simulink model "EPT"  (R2019b)
settings: Solver=FixedStepDiscrete  StartTime=0.0  StopTime=5  FixedStep=0.005  RelTol=1e-3  EnableMultiTasking=on
PreLoadFcn:
  | try, model_open; catch, disp('Error occurred while executing model pre-load callback: model_open.m'); disp('Please assure that the MATLAB working directory is set to the model directory before opening.'); end
InitFcn:
  | try, model_open; catch, end
undefined symbols (not defined in the file or in its folder): Bridge, GCM, H, ln, raptor_get_param_eval, raptor_get_safe_string, raptor_xcp_function
libraries: Raptor_lib x2810, simulink x374, hdlsllib x19
(part 1 of 45)
CloseFcn:
  | try, model_close; catch, end
settings Model: Raptor_Target=GCM-1793-196-1503  Raptor_Calloc=NonVolatile (EEPROM)  RaptorUIDSize=4  RaptorBuildNum=718  Raptor_ecuaddr=11  Raptor_IsLiteMode=0  Raptor_Redundant_NV=off  Raptor_Redundant_FNV=off  Creator=Ben  LastModifiedBy=user
settings SolverCC: AlgebraicLoopSolver=LineSearch
settings DataIOCC: LimitDataPoints=on  SaveFormat=Array  ReturnWorkspaceOutputs=off
settings OptimizationCC: DefaultParameterBehavior=Inlined  ExpressionDepthLimit=2147483647  InitFltsAndDblsToZero=on  LifeSpan=1  EfficientTunableParamExpr=on
settings DebuggingCC: SolverPrmCheckMsg=warning  InheritedTsInSrcMsg=none  FcnCallInpInsideContextMsg=warning  StateNameClashWarn=warning  SFUnexpectedBacktrackingDiag=warning  SFNoUnconditionalDefaultTransitionDiag=warning  SFExecutionAtInitializationDiag=none  ArithmeticOperatorsInVariantConditions=warning
settings HardwareCC: ProdBitPerPointer=32  ProdBitPerSizeT=32  ProdBitPerPtrDiffT=32  ProdLargestAtomicFloat=None  ProdWordSize=32  ProdHWDeviceType=Infineon->TriCore  TargetIntDivRoundTo=Zero  TargetEndianess=LittleEndian  ProdEqTarget=off
settings ModelReferenceCC: PropagateSignalLabelsOutOfModel=off
settings SFSimCC: SimUseLocalCustomCode=off  MATLABDynamicMemAlloc=off  CustomCodeUndefinedFunction=UseInterfaceOnly
settings RTWCC: Description=Raptor (tm)  SystemTargetFile=raptor.tlc  GenCodeOnly=on  MakeCommand=raptor_make_rtw  TemplateMakefile=raptor.tmf  RTWUseLocalCustomCode=off
settings CodeAppCC: IgnoreCustomStorageClasses=off  MaxIdLength=100  CustomSymbolStrType=$N$R$M  StateflowObjectComments=on  InternalIdentifier=Classic
settings STFCustomTargetCC: GenerateSampleERTMain=on  ModelReferenceCompliant=off  CombineOutputUpdateFcns=on  ERTCustomFileBanners=on  SupportContinuousTime=off  SupportNonInlinedSFcns=off  RemoveResetFunc=on  MATLABClassNameForMDSCustomization=Simulink.SoftwareTarget.ERTCustomization  SystemTargetFile=raptor.tlc
settings ERTTargetCC: MultiwordLength=2048  GenerateSampleERTMain=on  ModelReferenceCompliant=off  ParMdlRefBuildCompliant=off  CompOptLevelCompliant=off  ConcurrentExecutionCompliant=off  ModelStepFunctionPrototypeControlCompliant=off  CPPClassGenCompliant=off  UseToolchainInfoCompliant=off  ExtModeMexFile=noextcomm  InlinedParameterPlacement=NonHierarchical  ERTCustomFileTemplate=example_file_process.tlc  ConvertIfToSwitch=off  SuppressUnreachableDefaultCases=off
settings ConfigComp: CovMetricSettings=dw  CovHtmlReporting=on  CovSaveCumulativeToWorkspaceVar=on  CovSaveSingleToWorkspaceVar=on  CovExternalEMLEnable=off  CovSFcnEnable=off

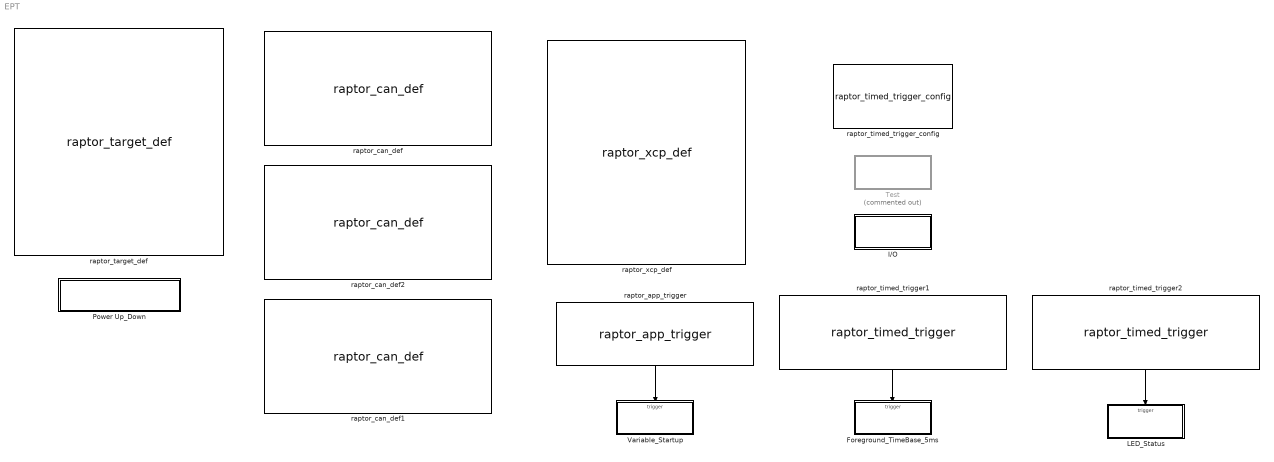
== system EPT ==
  Foreground_TimeBase_5ms : Subsystem  TreatAsAtomicUnit=on
      settings: RTWSystemCode=Nonreusable function
  I/O : Subsystem
  LED_Status : Subsystem  TreatAsAtomicUnit=on
      settings: RTWSystemCode=Nonreusable function
  Power Up_Down : Subsystem  mask{group='Diagnostics | Power Up_Down'}
  Test : Subsystem  Commented=on
  Variable_Startup : Subsystem  TreatAsAtomicUnit=on
      settings: RTWSystemCode=Nonreusable function
  raptor_app_trigger : Raptor_lib/Triggers/raptor_app_trigger  triggerValues=Startup|Shutdown|SafetyMonitor  trigger=Startup  inherited=0  alwaysEnabled=1  triggerPriority=0  triggerName=Startup_zGoy_  allowInline=0
      settings: SourceProductName=Raptor
  raptor_can_def : Raptor_lib/CAN/raptor_can_def  canBus='CAN1'  resourceValues=CAN1|CAN2|CAN3|(None)  resource=CAN1  baudRateValues=125k|250k|500k|1000k  baudRate=500k  txQueueSize=16  rxQueueSize=16
      settings: SourceProductName=Raptor
  raptor_can_def1 : Raptor_lib/CAN/raptor_can_def  canBus='CAN3'  resourceValues=CAN1|CAN2|CAN3|(None)  resource=CAN3  baudRateValues=125k|250k|500k|1000k  baudRate=500k  txQueueSize=16  rxQueueSize=16
      settings: SourceProductName=Raptor
  raptor_can_def2 : Raptor_lib/CAN/raptor_can_def  canBus='CAN2'  resourceValues=CAN1|CAN2|CAN3|(None)  resource=CAN2  baudRateValues=125k|250k|500k|1000k  baudRate=500k  txQueueSize=16  rxQueueSize=16
      settings: SourceProductName=Raptor
  raptor_target_def : Raptor_lib/Configuration/raptor_target_def  targetValues=BCM-5646-48-1404|DISP-VC128-1901|DISP-VC320L-1402|DISP-VC320-1204|DISP-VC800-1402|DISP-VC500-1904|GCM-5634M-070-1459|GCM-5634M-070-1559|GCM-5634M-070-1562|ECM-1793-196-1503|GCM-1793-196-1503|GCM-5607B-80-1901|GCM-5746R-048-1902|HCM-5534-50-1203|HCM-5534-90-1201|HCM-5534-90-1302|HCM-5534-90-1601|HCM-5534-90-1602|HCM-5604-36-1303|HCM-5604-36-1702|HCM-ARM4-070-1401|HCM-ARM4-070-1601  target=GCM-1793-196-1503  simpack=0  simulator=0  heap=4*1024  stack=2*1024  fgndStack=3*1024  bgndStack=2*1024  idleStack=1024  intStack=1536  sdStack=1024  appStack=1024  ecuaddr=11  callocValues=Constant (FLASH)|NonVolatile (EEPROM)  calloc=NonVolatile (EEPROM)  compilerValues=HighTec v3.4.5.11|HighTec v3.4.5.9  compiler=HighTec v3.4.5.11  setFileName=0  exeName=[raptor_get_safe_string(bdroot) '_']  addBuildNum=1  minVerChars=3  extraOutput=0  buildLocationValues=Raptor Default|Model Directory|User Defined  buildLocation=Raptor Default  exeLocation=''  a2lLocation=''  rpgLocation=''
      settings: SourceProductName=Raptor
  raptor_timed_trigger1 : Raptor_lib/Triggers/raptor_timed_trigger  triggerValues=Foreground|Foregroundx2|Foregroundx5|Foregroundx10|Foregroundx20|Background|Backgroundx2|Backgroundx5|Backgroundx10|Backgroundx20|Second|Minute  trigger=Foreground  inherited=0  alwaysEnabled=0  triggerPriority=0  triggerName=FGND_QFJFi
      settings: SourceProductName=Raptor
  raptor_timed_trigger2 : Raptor_lib/Triggers/raptor_timed_trigger  triggerValues=Foreground|Foregroundx2|Foregroundx5|Foregroundx10|Foregroundx20|Background|Backgroundx2|Backgroundx5|Backgroundx10|Backgroundx20|Second|Minute  trigger=Foreground  inherited=0  alwaysEnabled=0  triggerPriority=0  triggerName=FGND__22F5
      settings: SourceProductName=Raptor
  raptor_timed_trigger_config : Raptor_lib/Triggers/raptor_timed_trigger_config  triggerValues=Foreground|Background|Second|Minute  trigger=Foreground  period=5  CM2115newPeriod='RAPTOR MASK DEFAULT'
      settings: SourceProductName=Raptor
  raptor_xcp_def : Raptor_lib/Configuration/raptor_xcp_def  canBus='CAN1'  bcID=hex2dec('100')  bcID_TypeValues=Standard|Extended  bcID_Type=Standard  rxID=hex2dec('201')  rxID_TypeValues=Standard|Extended  rxID_Type=Standard  txID=hex2dec('301')  txID_TypeValues=Standard|Extended  txID_Type=Standard  daqRates=[5 10 100]  numODTs=20  genCANAPE=0  genVISION=0  securityValues=Standard|None|Custom User Defined  security=Standard  dllName=raptor_XCPSecurity.dll  accessValues=4|3|2|1  access=1
      settings: SourceProductName=Raptor
  wires:
  raptor_timed_trigger1/1 -> Foreground_TimeBase_5ms/Trigger
  raptor_app_trigger/1 -> Variable_Startup/Trigger
  raptor_timed_trigger2/1 -> LED_Status/Trigger

== system EPT/Foreground_TimeBase_5ms ==
  function : TriggerPort  TriggerType=function-call  VariantControl=Variant
  CAN : Subsystem
  CHG/DCHG_PW_Control : Subsystem
  Delay : Subsystem
  "E/W " : Subsystem
  Internal_Measurement : Subsystem
  NOT : Logic  Operator=NOT  IconShape=distinctive  AllPortsSameDT=off  OutDataTypeStr=boolean
  NOT1 : Logic  Operator=NOT  IconShape=distinctive  AllPortsSameDT=off  OutDataTypeStr=boolean
  OBP_Temp_Detection : Subsystem
  Oil/Water/Pack Cooling System : Subsystem
  System Initial : Subsystem
  System Setup : Subsystem
  SystemStart : Subsystem  TreatAsAtomicUnit=on
  raptor_adjustment8 : Raptor_lib/Data Storage/raptor_adjustment  paramName='Cal_Delay_System_Work'  nameSource=Parameter  initValue=1000  dataType=Inherit via back propagation  storage=Calibration  calDispType=Number  calEnum={'False', 'True'}  calGain=1.0  calOffset=0.0  calMax=inf  calMin=-inf  calFormat='-1'  calUnit=''  calHelp=''  calAccess=1  calFunction=raptor_xcp_function(gcb)  calDispHeaders=off  calColHeaders={'Col1' 'Col2' 'Col3'}  calRowHeaders={'Row1' 'Row2' 'Row3'}
      settings: SourceProductName=Raptor
  raptor_data_read1 : Raptor_lib/Data Storage/raptor_data_read  dataName='Flag_Ign_Off'  dataShape=Scalar  idxSource=Input  idxRow=1  idxCol=1
      settings: SourceProductName=Raptor
  raptor_data_read4 : Raptor_lib/Data Storage/raptor_data_read  dataName='Flag_Ign_Off'  dataShape=Scalar  idxSource=Input  idxRow=1  idxCol=1
      settings: SourceProductName=Raptor
  wires:
  raptor_data_read4/1 -> NOT/1
  raptor_adjustment8/1 -> Delay/2(TimeCount)
  Delay/1(Output) -> SystemStart/Trigger
  NOT/1 -> Delay/1(Condition)
  raptor_data_read1/1 -> NOT1/1, System Initial/Enable
  NOT1/1 -> CHG/DCHG_PW_Control/Enable, System Setup/Enable

== system EPT/I//O ==
  Application : Subsystem
  Input : Subsystem
  Output : Subsystem

== system EPT/LED_Status ==
  function : TriggerPort  TriggerType=function-call  VariantControl=Variant
  DualLED_Funny : Subsystem

== system EPT/Power Up_Down ==
  Background : Subsystem
  raptor_timed_trigger : Raptor_lib/Triggers/raptor_timed_trigger  triggerValues=Foreground|Foregroundx2|Foregroundx5|Foregroundx10|Foregroundx20|Background|Backgroundx2|Backgroundx5|Backgroundx10|Backgroundx20|Second|Minute  trigger=Background  inherited=0  alwaysEnabled=1  triggerPriority=50  triggerName=BGND_f_UiI
      settings: SourceProductName=Raptor
  wires:
  raptor_timed_trigger/1 -> Background/Trigger

== system EPT/Test ==
  Adjustment Variable : Subsystem  Commented=on
  Coulomb Counting Method Test : Subsystem  Commented=on
  DualLEDTest : Subsystem  Commented=on
  LED For CMU : Subsystem  Commented=on
  LifeCycleTest : Subsystem  Commented=on
  RPB1600_Read : Subsystem  Commented=on
  SINE_Wave : Subsystem  Commented=on
  Subsystem : Subsystem  Commented=on

== system EPT/Variable_Startup ==
  function : TriggerPort  TriggerType=function-call  VariantControl=Variant
  EEPROM Init : Subsystem
  Fault_init : Subsystem

== system EPT/Foreground_TimeBase_5ms/CAN ==
  CAN1_exec : Subsystem
  CAN2_exec : Subsystem
  CAN3_exec : Subsystem

== system EPT/Foreground_TimeBase_5ms/CHG//DCHG_PW_Control ==
  note: Notes:
      | IVT		:0
      | CMU	:1
  Enable : EnablePort  StatesWhenEnabling=reset
  Add : Sum
  Add1 : Sum
  Batt_Temperature Coefficient : Subsystem
  CHG/DCHG_Current_Control : Subsystem
  Coulomb Counting Algorithm : Subsystem
  Data Type Conversion{,1..3} (4 alike) : DataTypeConversion
  Demux : Demux  Outputs=2
  EOC : Subsystem
  EOD : Subsystem
  Enhanced Coulomb Counting Algorithm : Subsystem  Commented=on
  Enhanced Coulomb Counting Algorithm Backup : Subsystem  Commented=on
  Gain1 : Gain  Gain=0.5
  Gain2 : Gain  Gain=-1
  Maximum allowable Regen torque : Subsystem
  Maximum allowable torque : Subsystem
  Mux : Mux  Inputs=2
  Mux1 : Mux  Inputs=2
  PWCU PW Requirement : Subsystem
  SWU Power Divider : Subsystem
  Switch : Switch  Criteria=u2 > Threshold
  raptor_adjustment : Raptor_lib/Data Storage/raptor_adjustment  paramName='Cal_HV_DataSource'  nameSource=Parameter  initValue=0.00  dataType=double  storage=Calibration  calDispType=Number  calEnum={'False', 'True'}  calGain=1.0  calOffset=0.0  calMax=inf  calMin=-inf  calFormat='-1'  calUnit=''  calHelp=''  calAccess=1  calFunction=raptor_xcp_function(gcb)  calDispHeaders=off  calColHeaders={'Col1' 'Col2' 'Col3'}  calRowHeaders={'Row1' 'Row2' 'Row3'}
      settings: SourceProductName=Raptor
  raptor_data_def : Raptor_lib/Data Storage/raptor_data_def  dataName='EPT_BPOBU_SOC'  initValue=0  dataType=double  storage=Calibration  calVisible=on  calType=Measurement  calDispType=Number  calEnum={'False', 'True'}  calGain=1.0  calOffset=0  calMin=-inf  calMax=100  calFormat='-1'  calUnit=''  calHelp=''  calAccess=1  calFunction=raptor_xcp_function(gcb)  calDispHeaders=off  calColHeaders={'Col1' 'Col2' 'Col3'}  calRowHeaders={'Row1' 'Row2' 'Row3'}
      settings: SourceProductName=Raptor
  raptor_data_def1 : Raptor_lib/Data Storage/raptor_data_def  dataName='EPT_BPOBU_FCCAP'  initValue=0  dataType=double  storage=Volatile (RAM)  calVisible=on  calType=Measurement  calDispType=Number  calEnum={'False', 'True'}  calGain=1.0  calOffset=0  calMin=-inf  calMax=inf  calFormat='-1'  calUnit=''  calHelp=''  calAccess=1  calFunction=raptor_xcp_function(gcb)  calDispHeaders=off  calColHeaders={'Col1' 'Col2' 'Col3'}  calRowHeaders={'Row1' 'Row2' 'Row3'}
      settings: SourceProductName=Raptor
  raptor_data_def10 : Raptor_lib/Data Storage/raptor_data_def  dataName='Delta_DOD'  initValue=0  dataType=double  storage=Volatile (RAM)  calVisible=on  calType=Measurement  calDispType=Number  calEnum={'False', 'True'}  calGain=1.0  calOffset=0  calMin=-inf  calMax=inf  calFormat='-1'  calUnit=''  calHelp=''  calAccess=1  calFunction=raptor_xcp_function(gcb)  calDispHeaders=off  calColHeaders={'Col1' 'Col2' 'Col3'}  calRowHeaders={'Row1' 'Row2' 'Row3'}
      settings: SourceProductName=Raptor
  raptor_data_def11 : Raptor_lib/Data Storage/raptor_data_def  dataName='Cmax'  initValue=0  dataType=double  storage=Volatile (RAM)  calVisible=on  calType=Measurement  calDispType=Number  calEnum={'False', 'True'}  calGain=1.0  calOffset=0  calMin=-inf  calMax=inf  calFormat='-1'  calUnit=''  calHelp=''  calAccess=1  calFunction=raptor_xcp_function(gcb)  calDispHeaders=off  calColHeaders={'Col1' 'Col2' 'Col3'}  calRowHeaders={'Row1' 'Row2' 'Row3'}
      settings: SourceProductName=Raptor
  raptor_data_def12 : Raptor_lib/Data Storage/raptor_data_def  dataName='SOC'  initValue=0  dataType=double  storage=Volatile (RAM)  calVisible=on  calType=Measurement  calDispType=Number  calEnum={'False', 'True'}  calGain=1.0  calOffset=0  calMin=-inf  calMax=inf  calFormat='-1'  calUnit=''  calHelp=''  calAccess=1  calFunction=raptor_xcp_function(gcb)  calDispHeaders=off  calColHeaders={'Col1' 'Col2' 'Col3'}  calRowHeaders={'Row1' 'Row2' 'Row3'}
      settings: SourceProductName=Raptor
  raptor_data_def13 : Raptor_lib/Data Storage/raptor_data_def  dataName='SOH'  initValue=100  dataType=double  storage=Volatile (RAM)  calVisible=on  calType=Measurement  calDispType=Number  calEnum={'False', 'True'}  calGain=1.0  calOffset=0  calMin=-inf  calMax=inf  calFormat='-1'  calUnit=''  calHelp=''  calAccess=1  calFunction=raptor_xcp_function(gcb)  calDispHeaders=off  calColHeaders={'Col1' 'Col2' 'Col3'}  calRowHeaders={'Row1' 'Row2' 'Row3'}
      settings: SourceProductName=Raptor
  raptor_data_def14 : Raptor_lib/Data Storage/raptor_data_def  dataName='EPT_BPOBU_VOLT'  initValue=0  dataType=double  storage=Calibration  calVisible=on  calType=Measurement  calDispType=Number  calEnum={'False', 'True'}  calGain=1.0  calOffset=0  calMin=-inf  calMax=inf  calFormat='-1'  calUnit=''  calHelp=''  calAccess=1  calFunction=raptor_xcp_function(gcb)  calDispHeaders=off  calColHeaders={'Col1' 'Col2' 'Col3'}  calRowHeaders={'Row1' 'Row2' 'Row3'}
      settings: SourceProductName=Raptor
  raptor_data_def15 : Raptor_lib/Data Storage/raptor_data_def  dataName='DOD_t'  initValue=0  dataType=double  storage=Volatile (RAM)  calVisible=on  calType=Measurement  calDispType=Number  calEnum={'False', 'True'}  calGain=1.0  calOffset=0  calMin=-inf  calMax=inf  calFormat='-1'  calUnit=''  calHelp=''  calAccess=1  calFunction=raptor_xcp_function(gcb)  calDispHeaders=off  calColHeaders={'Col1' 'Col2' 'Col3'}  calRowHeaders={'Row1' 'Row2' 'Row3'}
      settings: SourceProductName=Raptor
  raptor_data_def2 : Raptor_lib/Data Storage/raptor_data_def  dataName='EPT_HV_BUS_VOLT'  initValue=0  dataType=double  storage=Calibration  calVisible=on  calType=Measurement  calDispType=Number  calEnum={'False', 'True'}  calGain=1.0  calOffset=0  calMin=-inf  calMax=inf  calFormat='-1'  calUnit=''  calHelp=''  calAccess=1  calFunction=raptor_xcp_function(gcb)  calDispHeaders=off  calColHeaders={'Col1' 'Col2' 'Col3'}  calRowHeaders={'Row1' 'Row2' 'Row3'}
      settings: SourceProductName=Raptor
  raptor_data_def3 : Raptor_lib/Data Storage/raptor_data_def  dataName='EPT_BPOBU_AH_DEF'  initValue=0  dataType=uint8  storage=Volatile (RAM)  calVisible=on  calType=Measurement  calDispType=Number  calEnum={'False', 'True'}  calGain=1.0  calOffset=0  calMin=-inf  calMax=inf  calFormat='-1'  calUnit=''  calHelp=''  calAccess=1  calFunction=raptor_xcp_function(gcb)  calDispHeaders=off  calColHeaders={'Col1' 'Col2' 'Col3'}  calRowHeaders={'Row1' 'Row2' 'Row3'}
      settings: SourceProductName=Raptor
  raptor_data_def4 : Raptor_lib/Data Storage/raptor_data_def  dataName='EPT_BPOBU_RCAP'  initValue=0  dataType=double  storage=Volatile (RAM)  calVisible=on  calType=Measurement  calDispType=Number  calEnum={'False', 'True'}  calGain=1.0  calOffset=0  calMin=-inf  calMax=150  calFormat='-1'  calUnit=''  calHelp=''  calAccess=1  calFunction=raptor_xcp_function(gcb)  calDispHeaders=off  calColHeaders={'Col1' 'Col2' 'Col3'}  calRowHeaders={'Row1' 'Row2' 'Row3'}
      settings: SourceProductName=Raptor
  raptor_data_def5 : Raptor_lib/Data Storage/raptor_data_def  dataName='EPT_BPOBU_SOA'  initValue=1  dataType=double  storage=Volatile (RAM)  calVisible=on  calType=Measurement  calDispType=Number  calEnum={'False', 'True'}  calGain=1.0  calOffset=0  calMin=-inf  calMax=inf  calFormat='-1'  calUnit=''  calHelp=''  calAccess=1  calFunction=raptor_xcp_function(gcb)  calDispHeaders=off  calColHeaders={'Col1' 'Col2' 'Col3'}  calRowHeaders={'Row1' 'Row2' 'Row3'}
      settings: SourceProductName=Raptor
  raptor_data_def6 : Raptor_lib/Data Storage/raptor_data_def  dataName='EPT_HV_LEAK_VOLT'  initValue=0  dataType=double  storage=Calibration  calVisible=on  calType=Measurement  calDispType=Number  calEnum={'False', 'True'}  calGain=1.0  calOffset=0  calMin=-inf  calMax=inf  calFormat='-1'  calUnit=''  calHelp=''  calAccess=1  calFunction=raptor_xcp_function(gcb)  calDispHeaders=off  calColHeaders={'Col1' 'Col2' 'Col3'}  calRowHeaders={'Row1' 'Row2' 'Row3'}
      settings: SourceProductName=Raptor
  raptor_data_def7 : Raptor_lib/Data Storage/raptor_data_def  dataName='EPT_BPOBU_CURR'  initValue=0  dataType=double  storage=Calibration  calVisible=on  calType=Measurement  calDispType=Number  calEnum={'False', 'True'}  calGain=1.0  calOffset=0  calMin=-inf  calMax=inf  calFormat='-1'  calUnit=''  calHelp=''  calAccess=1  calFunction=raptor_xcp_function(gcb)  calDispHeaders=off  calColHeaders={'Col1' 'Col2' 'Col3'}  calRowHeaders={'Row1' 'Row2' 'Row3'}
      settings: SourceProductName=Raptor
  raptor_data_def8 : Raptor_lib/Data Storage/raptor_data_def  dataName='New_SOH'  initValue=100  dataType=double  storage=Volatile (RAM)  calVisible=on  calType=Measurement  calDispType=Number  calEnum={'False', 'True'}  calGain=1.0  calOffset=0  calMin=-inf  calMax=inf  calFormat='-1'  calUnit=''  calHelp=''  calAccess=1  calFunction=raptor_xcp_function(gcb)  calDispHeaders=off  calColHeaders={'Col1' 'Col2' 'Col3'}  calRowHeaders={'Row1' 'Row2' 'Row3'}
      settings: SourceProductName=Raptor
  raptor_data_def9 : Raptor_lib/Data Storage/raptor_data_def  dataName='DOD_t0'  initValue=0  dataType=double  storage=Volatile (RAM)  calVisible=on  calType=Measurement  calDispType=Number  calEnum={'False', 'True'}  calGain=1.0  calOffset=0  calMin=-inf  calMax=inf  calFormat='-1'  calUnit=''  calHelp=''  calAccess=1  calFunction=raptor_xcp_function(gcb)  calDispHeaders=off  calColHeaders={'Col1' 'Col2' 'Col3'}  calRowHeaders={'Row1' 'Row2' 'Row3'}
      settings: SourceProductName=Raptor
  raptor_data_read1 : Raptor_lib/Data Storage/raptor_data_read  dataName='CMU2_BATT_CURR'  dataShape=Scalar  idxSource=Input  idxRow=1  idxCol=1
      settings: SourceProductName=Raptor
  raptor_data_read10 : Raptor_lib/Data Storage/raptor_data_read  dataName='I_Current'  dataShape=Scalar  idxSource=Input  idxRow=1  idxCol=1
      settings: SourceProductName=Raptor
  raptor_data_read11 : Raptor_lib/Data Storage/raptor_data_read  dataName='U1_Voltage'  dataShape=Scalar  idxSource=Input  idxRow=1  idxCol=1
      settings: SourceProductName=Raptor
  raptor_data_read12 : Raptor_lib/Data Storage/raptor_data_read  dataName='U2_Voltage'  dataShape=Scalar  idxSource=Input  idxRow=1  idxCol=1
      settings: SourceProductName=Raptor
  raptor_data_read13 : Raptor_lib/Data Storage/raptor_data_read  dataName='U3_Voltage'  dataShape=Scalar  idxSource=Input  idxRow=1  idxCol=1
      settings: SourceProductName=Raptor
  raptor_data_read2 : Raptor_lib/Data Storage/raptor_data_read  dataName='CMU1_BATT_CURR'  dataShape=Scalar  idxSource=Input  idxRow=1  idxCol=1
      settings: SourceProductName=Raptor
  raptor_data_read4 : Raptor_lib/Data Storage/raptor_data_read  dataName='CMU2_BATT_VOLT'  dataShape=Scalar  idxSource=Input  idxRow=1  idxCol=1
      settings: SourceProductName=Raptor
  raptor_data_read7 : Raptor_lib/Data Storage/raptor_data_read  dataName='CMU1_BATT_VOLT'  dataShape=Scalar  idxSource=Input  idxRow=1  idxCol=1
      settings: SourceProductName=Raptor
  raptor_data_write1 : Raptor_lib/Data Storage/raptor_data_write  dataName='EPT_BPOBU_CURR'  dataShape=Scalar  idxSource=Input Port  idxRow=1  idxCol=1
      settings: SourceProductName=Raptor
  raptor_data_write2 : Raptor_lib/Data Storage/raptor_data_write  dataName='EPT_BPOBU_VOLT'  dataShape=Scalar  idxSource=Input Port  idxRow=1  idxCol=1
      settings: SourceProductName=Raptor
  raptor_data_write4 : Raptor_lib/Data Storage/raptor_data_write  dataName='EPT_HV_BUS_VOLT'  dataShape=Scalar  idxSource=Input Port  idxRow=1  idxCol=1
      settings: SourceProductName=Raptor
  raptor_data_write5 : Raptor_lib/Data Storage/raptor_data_write  dataName='EPT_HV_LEAK_VOLT'  dataShape=Scalar  idxSource=Input Port  idxRow=1  idxCol=1
      settings: SourceProductName=Raptor
  wires:
  Batt_Temperature Coefficient/1(Ft) -> CHG/DCHG_Current_Control/1(Ft)
  raptor_data_read4/1 -> Add/2
  raptor_data_read7/1 -> Add/1
  CHG/DCHG_Current_Control/1(Idchg_exp) -> Maximum allowable torque/1(Idchg_con)
  Add1/1 -> Gain1/1
  raptor_data_read2/1 -> Add1/1
  raptor_data_read1/1 -> Add1/2
  CHG/DCHG_Current_Control/2(Iregen_con) -> Maximum allowable Regen torque/1(Iregen_con)
  Mux/1 -> Switch/3
  raptor_data_read10/1 -> Data Type Conversion/1
  raptor_data_read11/1 -> Data Type Conversion1/1
  Switch/1 -> Demux/1
  Gain1/1 -> Mux1/1
  Add/1 -> Mux1/2
  Mux1/1 -> Switch/1
  Demux/1 -> raptor_data_write1/1
  Demux/2 -> raptor_data_write2/1
  Data Type Conversion/1 -> Gain2/1
  Data Type Conversion1/1 -> Mux/2
  raptor_adjustment/1 -> Switch/2
  raptor_data_read12/1 -> Data Type Conversion2/1
  raptor_data_read13/1 -> Data Type Conversion3/1
  Data Type Conversion2/1 -> raptor_data_write4/1
  Data Type Conversion3/1 -> raptor_data_write5/1
  Gain2/1 -> Mux/1

== system EPT/Foreground_TimeBase_5ms/Delay ==
  Condition : Inport
  TimeCount : Inport  Port=2
  Constant10 : Constant
  Constant11 : Constant  Value=0
  Constant8 : Constant  Value=0
  CycleTrigger : Subsystem
  Switch2 : Switch  Threshold=1
  Switch3 : Switch  Threshold=1
  Unit Delay1 : UnitDelay  SampleTime=-1  HasFrameUpgradeWarning=on
  Unit Delay3 : UnitDelay  SampleTime=-1  HasFrameUpgradeWarning=on
  Output : Outport  VectorParamsAs1DForOutWhenUnconnected=off
  wires:
  TimeCount/1 -> CycleTrigger/2(In2)
  Condition/1 -> Switch3/2
  Constant8/1 -> Switch2/1
  CycleTrigger/1(Trigger) -> Switch2/2, Unit Delay3/1
  Constant10/1 -> Switch2/3
  Switch3/1 -> CycleTrigger/1(In1)
  Switch2/1 -> Unit Delay1/1
  Constant11/1 -> Switch3/3
  Unit Delay1/1 -> Switch3/1
  Unit Delay3/1 -> Output/1

== system EPT/Foreground_TimeBase_5ms/E//W  ==
  BP-OBU_E/W : Subsystem
  CAN_E/W : Subsystem
  E/W_Process : Subsystem

== system EPT/Foreground_TimeBase_5ms/Internal_Measurement ==
  raptor_data_def1 : Raptor_lib/Data Storage/raptor_data_def  dataName='Sensor_5V_Volt'  initValue=0  dataType=double  storage=Volatile (RAM)  calVisible=on  calType=Measurement  calDispType=Number  calEnum={'False', 'True'}  calGain=1.0  calOffset=0  calMin=-inf  calMax=inf  calFormat='-1'  calUnit=''  calHelp=''  calAccess=1  calFunction=raptor_xcp_function(gcb)  calDispHeaders=off  calColHeaders={'Col1' 'Col2' 'Col3'}  calRowHeaders={'Row1' 'Row2' 'Row3'}
      settings: SourceProductName=Raptor
  raptor_data_def4 : Raptor_lib/Data Storage/raptor_data_def  dataName='I2V_Battery_Volt'  initValue=0  dataType=double  storage=Volatile (RAM)  calVisible=on  calType=Measurement  calDispType=Number  calEnum={'False', 'True'}  calGain=1.0  calOffset=0  calMin=-inf  calMax=inf  calFormat='-1'  calUnit=''  calHelp=''  calAccess=1  calFunction=raptor_xcp_function(gcb)  calDispHeaders=off  calColHeaders={'Col1' 'Col2' 'Col3'}  calRowHeaders={'Row1' 'Row2' 'Row3'}
      settings: SourceProductName=Raptor
  raptor_data_write1 : Raptor_lib/Data Storage/raptor_data_write  dataName='Sensor_5V_Volt'  dataShape=Scalar  idxSource=Input Port  idxRow=1  idxCol=1
      settings: SourceProductName=Raptor
  raptor_data_write2 : Raptor_lib/Data Storage/raptor_data_write  dataName='I2V_Battery_Volt'  dataShape=Scalar  idxSource=Input Port  idxRow=1  idxCol=1
      settings: SourceProductName=Raptor
  raptor_internal_measurement : Raptor_lib/Input & Output/raptor_internal_measurement  resourceValues=BATTERY_VOLTAGE|VSENS_SUPPLY|LAST_RESET|RESET_CNT|(None)  resource=BATTERY_VOLTAGE  out_eng=1  soft_filter=1  out_bool=0
      settings: SourceProductName=Raptor
  raptor_internal_measurement1 : Raptor_lib/Input & Output/raptor_internal_measurement  resourceValues=BATTERY_VOLTAGE|VSENS_SUPPLY|LAST_RESET|RESET_CNT|(None)  resource=VSENS_SUPPLY  out_eng=1  soft_filter=1  out_bool=0
      settings: SourceProductName=Raptor
  raptor_internal_measurement2 : Raptor_lib/Input & Output/raptor_internal_measurement  resourceValues=BATTERY_VOLTAGE|VSENS_SUPPLY|LAST_RESET|RESET_CNT|(None)  resource=LAST_RESET  out_eng=1  soft_filter=1  out_bool=0
      settings: SourceProductName=Raptor
  raptor_internal_measurement3 : Raptor_lib/Input & Output/raptor_internal_measurement  resourceValues=BATTERY_VOLTAGE|VSENS_SUPPLY|LAST_RESET|RESET_CNT|(None)  resource=RESET_CNT  out_eng=1  soft_filter=1  out_bool=0
      settings: SourceProductName=Raptor
  raptor_measurement2 : Raptor_lib/Data Storage/raptor_measurement  paramName='Last_Reset'  nameSource=Parameter  calDispType=Number  calEnum={'False', 'True'}  calGain=1.0  calOffset=0.0  calMax=inf  calMin=-inf  calFormat='-1'  calUnit=''  calHelp=''  calAccess=1  calFunction=raptor_xcp_function(gcb)  calVisible=on
      settings: SourceProductName=Raptor
  raptor_measurement3 : Raptor_lib/Data Storage/raptor_measurement  paramName='Reset_CNT'  nameSource=Parameter  calDispType=Number  calEnum={'False', 'True'}  calGain=1.0  calOffset=0.0  calMax=inf  calMin=-inf  calFormat='-1'  calUnit=''  calHelp=''  calAccess=1  calFunction=raptor_xcp_function(gcb)  calVisible=on
      settings: SourceProductName=Raptor
  wires:
  raptor_internal_measurement/1 -> raptor_data_write2/1
  raptor_internal_measurement3/1 -> raptor_measurement3/1
  raptor_internal_measurement2/1 -> raptor_measurement2/1
  raptor_internal_measurement1/1 -> raptor_data_write1/1

== system EPT/Foreground_TimeBase_5ms/OBP_Temp_Detection ==
  ADC2Degree : Subsystem
  Constant2 : Constant  Value=20
  CountTrigger : Subsystem
  wires:
  CountTrigger/1(Tirgger) -> ADC2Degree/Trigger
  Constant2/1 -> CountTrigger/1(Counter)

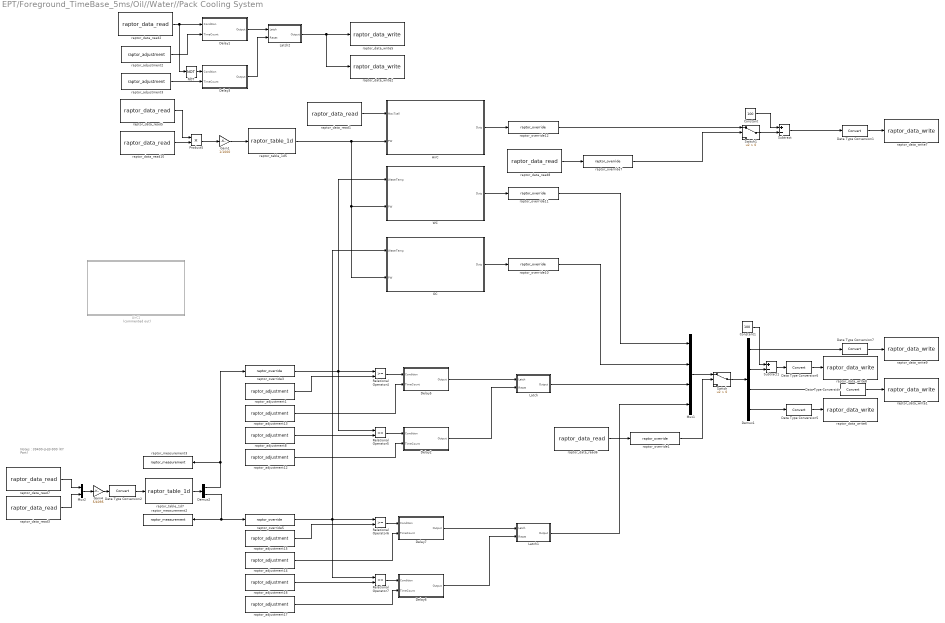
== system EPT/Foreground_TimeBase_5ms/Oil//Water//Pack Cooling System ==
  note: Notes :
      | 39400-LHJ3-900
      | (KY Part)
  AirC : Subsystem
  AirC1 : Subsystem  Commented=on
  Constant : Constant  Value=100
  Constant1 : Constant  Value=100
  Data Type Conversion{,1..2,5..7} (6 alike) : DataTypeConversion
  Delay1 : Subsystem
  Delay2 : Subsystem
  Delay3 : Subsystem
  Delay5 : Subsystem
  Delay6 : Subsystem
  Delay7 : Subsystem
  Demux1 : Demux
  Demux2 : Demux  Outputs=2
  Gain1 : Gain  Gain=1/1000
  Gain4 : Gain  Gain=5/4095
  Latch : Subsystem
  Latch1 : Subsystem
  Latch2 : Subsystem
  Mux1 : Mux
  Mux2 : Mux  Inputs=2
  NOT : Logic  Operator=NOT  IconShape=distinctive  AllPortsSameDT=off  OutDataTypeStr=boolean
  OC : Subsystem
  Product5 : Product
  Relational Operator4 : RelationalOperator  OutDataTypeStr=boolean  RndMeth=Simplest
  Relational Operator5 : RelationalOperator  Operator=<=  OutDataTypeStr=boolean  RndMeth=Simplest
  Relational Operator6 : RelationalOperator  OutDataTypeStr=boolean  RndMeth=Simplest
  Relational Operator7 : RelationalOperator  Operator=<=  OutDataTypeStr=boolean  RndMeth=Simplest
  Subtract : Sum  Inputs=+-
  Subtract1 : Sum  Inputs=+-
  Switch : Switch  Criteria=u2 > Threshold
  Switch1 : Switch  Criteria=u2 > Threshold
  WC : Subsystem
  raptor_adjustment1 : Raptor_lib/Data Storage/raptor_adjustment  paramName='Cal_Cooling_Water_Temp_LimitHigh'  nameSource=Parameter  initValue=55  dataType=double  storage=Calibration  calDispType=Number  calEnum={'False', 'True'}  calGain=1.0  calOffset=0.0  calMax=inf  calMin=-inf  calFormat='-1'  calUnit=''  calHelp=''  calAccess=1  calFunction=raptor_xcp_function(gcb)  calDispHeaders=off  calColHeaders={'Col1' 'Col2' 'Col3'}  calRowHeaders={'Row1' 'Row2' 'Row3'}
      settings: SourceProductName=Raptor
  raptor_adjustment12 : Raptor_lib/Data Storage/raptor_adjustment  paramName='Cal_Water_Cooling_Fan_Off_DelayTime'  nameSource=Parameter  initValue=1000  dataType=double  storage=Calibration  calDispType=Number  calEnum={'False', 'True'}  calGain=1.0  calOffset=0.0  calMax=inf  calMin=-inf  calFormat='-1'  calUnit=''  calHelp=''  calAccess=1  calFunction=raptor_xcp_function(gcb)  calDispHeaders=off  calColHeaders={'Col1' 'Col2' 'Col3'}  calRowHeaders={'Row1' 'Row2' 'Row3'}
      settings: SourceProductName=Raptor
  raptor_adjustment13 : Raptor_lib/Data Storage/raptor_adjustment  paramName='Cal_Water_Cooling_Fan_On_DelayTime'  nameSource=Parameter  initValue=0.00  dataType=double  storage=Calibration  calDispType=Number  calEnum={'False', 'True'}  calGain=1.0  calOffset=0.0  calMax=inf  calMin=-inf  calFormat='-1'  calUnit=''  calHelp=''  calAccess=1  calFunction=raptor_xcp_function(gcb)  calDispHeaders=off  calColHeaders={'Col1' 'Col2' 'Col3'}  calRowHeaders={'Row1' 'Row2' 'Row3'}
      settings: SourceProductName=Raptor
  raptor_adjustment14 : Raptor_lib/Data Storage/raptor_adjustment  paramName='Cal_Oil_Cooling_Fan_On_DelayTime'  nameSource=Parameter  initValue=0.00  dataType=double  storage=Calibration  calDispType=Number  calEnum={'False', 'True'}  calGain=1.0  calOffset=0.0  calMax=inf  calMin=-inf  calFormat='-1'  calUnit=''  calHelp=''  calAccess=1  calFunction=raptor_xcp_function(gcb)  calDispHeaders=off  calColHeaders={'Col1' 'Col2' 'Col3'}  calRowHeaders={'Row1' 'Row2' 'Row3'}
      settings: SourceProductName=Raptor
  raptor_adjustment15 : Raptor_lib/Data Storage/raptor_adjustment  paramName='Cal_Cooling_Oil_Temp_LimitHigh'  nameSource=Parameter  initValue=70  dataType=double  storage=Calibration  calDispType=Number  calEnum={'False', 'True'}  calGain=1.0  calOffset=0.0  calMax=inf  calMin=-inf  calFormat='-1'  calUnit=''  calHelp=''  calAccess=1  calFunction=raptor_xcp_function(gcb)  calDispHeaders=off  calColHeaders={'Col1' 'Col2' 'Col3'}  calRowHeaders={'Row1' 'Row2' 'Row3'}
      settings: SourceProductName=Raptor
  raptor_adjustment16 : Raptor_lib/Data Storage/raptor_adjustment  paramName='Cal_Cooling_Oil_Temp_LimitLow'  nameSource=Parameter  initValue=60  dataType=double  storage=Calibration  calDispType=Number  calEnum={'False', 'True'}  calGain=1.0  calOffset=0.0  calMax=inf  calMin=-inf  calFormat='-1'  calUnit=''  calHelp=''  calAccess=1  calFunction=raptor_xcp_function(gcb)  calDispHeaders=off  calColHeaders={'Col1' 'Col2' 'Col3'}  calRowHeaders={'Row1' 'Row2' 'Row3'}
      settings: SourceProductName=Raptor
  raptor_adjustment17 : Raptor_lib/Data Storage/raptor_adjustment  paramName='Cal_Oil_Cooling_Fan_Off_DelayTime'  nameSource=Parameter  initValue=3000  dataType=double  storage=Calibration  calDispType=Number  calEnum={'False', 'True'}  calGain=1.0  calOffset=0.0  calMax=inf  calMin=-inf  calFormat='-1'  calUnit=''  calHelp=''  calAccess=1  calFunction=raptor_xcp_function(gcb)  calDispHeaders=off  calColHeaders={'Col1' 'Col2' 'Col3'}  calRowHeaders={'Row1' 'Row2' 'Row3'}
      settings: SourceProductName=Raptor
  raptor_adjustment2 : Raptor_lib/Data Storage/raptor_adjustment  paramName='Cal_EAU_On_DelayTime'  nameSource=Parameter  initValue=0.00  dataType=double  storage=Calibration  calDispType=Number  calEnum={'False', 'True'}  calGain=1.0  calOffset=0.0  calMax=inf  calMin=-inf  calFormat='-1'  calUnit=''  calHelp=''  calAccess=1  calFunction=raptor_xcp_function(gcb)  calDispHeaders=off  calColHeaders={'Col1' 'Col2' 'Col3'}  calRowHeaders={'Row1' 'Row2' 'Row3'}
      settings: SourceProductName=Raptor
  raptor_adjustment3 : Raptor_lib/Data Storage/raptor_adjustment  paramName='Cal_EAU_Off_DelayTime'  nameSource=Parameter  initValue=100  dataType=double  storage=Calibration  calDispType=Number  calEnum={'False', 'True'}  calGain=1.0  calOffset=0.0  calMax=inf  calMin=-inf  calFormat='-1'  calUnit=''  calHelp=''  calAccess=1  calFunction=raptor_xcp_function(gcb)  calDispHeaders=off  calColHeaders={'Col1' 'Col2' 'Col3'}  calRowHeaders={'Row1' 'Row2' 'Row3'}
      settings: SourceProductName=Raptor
  raptor_adjustment8 : Raptor_lib/Data Storage/raptor_adjustment  paramName='Cal_Cooling_Water_Temp_LimitLow'  nameSource=Parameter  initValue=50  dataType=double  storage=Calibration  calDispType=Number  calEnum={'False', 'True'}  calGain=1.0  calOffset=0.0  calMax=inf  calMin=-inf  calFormat='-1'  calUnit=''  calHelp=''  calAccess=1  calFunction=raptor_xcp_function(gcb)  calDispHeaders=off  calColHeaders={'Col1' 'Col2' 'Col3'}  calRowHeaders={'Row1' 'Row2' 'Row3'}
      settings: SourceProductName=Raptor
  raptor_data_read1 : Raptor_lib/Data Storage/raptor_data_read  dataName='Max_CellT'  dataShape=Scalar  idxSource=Input  idxRow=1  idxCol=1
      settings: SourceProductName=Raptor
  raptor_data_read10 : Raptor_lib/Data Storage/raptor_data_read  dataName='EPT_BPOBU_VOLT'  dataShape=Scalar  idxSource=Input  idxRow=1  idxCol=1
      settings: SourceProductName=Raptor
  raptor_data_read2 : Raptor_lib/Data Storage/raptor_data_read  dataName='Relay_DCDC_12V'  dataShape=Scalar  idxSource=Input  idxRow=1  idxCol=1
      settings: SourceProductName=Raptor
  raptor_data_read3 : Raptor_lib/Data Storage/raptor_data_read  dataName='A105_Cooling_Oil_Temp_in'  dataShape=Scalar  idxSource=Input  idxRow=1  idxCol=1
      settings: SourceProductName=Raptor
  raptor_data_read5 : Raptor_lib/Data Storage/raptor_data_read  dataName='EPT_BPOBU_CURR'  dataShape=Scalar  idxSource=Input  idxRow=1  idxCol=1
      settings: SourceProductName=Raptor
  raptor_data_read6 : Raptor_lib/Data Storage/raptor_data_read  dataName='K37_LSD_Relay_EAU1'  dataShape=Scalar  idxSource=Input  idxRow=1  idxCol=1
      settings: SourceProductName=Raptor
  raptor_data_read7 : Raptor_lib/Data Storage/raptor_data_read  dataName='A17_Cooling_Water_Temp_in'  dataShape=Scalar  idxSource=Input  idxRow=1  idxCol=1
      settings: SourceProductName=Raptor
  raptor_data_read8 : Raptor_lib/Data Storage/raptor_data_read  dataName='K19_LSD_Relay_EAU2'  dataShape=Scalar  idxSource=Input  idxRow=1  idxCol=1
      settings: SourceProductName=Raptor
  raptor_data_write1 : Raptor_lib/Data Storage/raptor_data_write  dataName='K55_LSD_Relay_WC'  dataShape=Scalar  idxSource=Input Port  idxRow=1  idxCol=1
      settings: SourceProductName=Raptor
  raptor_data_write2 : Raptor_lib/Data Storage/raptor_data_write  dataName='K19_LSD_Relay_EAU2'  dataShape=Scalar  idxSource=Input Port  idxRow=1  idxCol=1
      settings: SourceProductName=Raptor
  raptor_data_write5 : Raptor_lib/Data Storage/raptor_data_write  dataName='K37_LSD_Relay_EAU1'  dataShape=Scalar  idxSource=Input Port  idxRow=1  idxCol=1
      settings: SourceProductName=Raptor
  raptor_data_write6 : Raptor_lib/Data Storage/raptor_data_write  dataName='A46_LSD_Relay_OC'  dataShape=Scalar  idxSource=Input Port  idxRow=1  idxCol=1
      settings: SourceProductName=Raptor
  raptor_data_write7 : Raptor_lib/Data Storage/raptor_data_write  dataName='K88_LSD_PWM_Duty'  dataShape=Scalar  idxSource=Input Port  idxRow=1  idxCol=1
      settings: SourceProductName=Raptor
  raptor_data_write8 : Raptor_lib/Data Storage/raptor_data_write  dataName='A23_LSD_PWM_Duty'  dataShape=Scalar  idxSource=Input Port  idxRow=1  idxCol=1
      settings: SourceProductName=Raptor
  raptor_data_write9 : Raptor_lib/Data Storage/raptor_data_write  dataName='A93_LSD_PWM_Duty'  dataShape=Scalar  idxSource=Input Port  idxRow=1  idxCol=1
      settings: SourceProductName=Raptor
  raptor_measurement2 : Raptor_lib/Data Storage/raptor_measurement  paramName='Oil_Temp'  nameSource=Parameter  calDispType=Number  calEnum={'False', 'True'}  calGain=1.0  calOffset=0.0  calMax=inf  calMin=-inf  calFormat='-1'  calUnit=''  calHelp=''  calAccess=1  calFunction=raptor_xcp_function(gcb)  calVisible=on
      settings: SourceProductName=Raptor
  raptor_measurement3 : Raptor_lib/Data Storage/raptor_measurement  paramName='Water_Temp'  nameSource=Parameter  calDispType=Number  calEnum={'False', 'True'}  calGain=1.0  calOffset=0.0  calMax=inf  calMin=-inf  calFormat='-1'  calUnit=''  calHelp=''  calAccess=1  calFunction=raptor_xcp_function(gcb)  calVisible=on
      settings: SourceProductName=Raptor
  raptor_override1 : Raptor_lib/Data Storage/raptor_override  paramName='Cal_Motor_Cooling_System_Output'  nameSource=Parameter  measurement=None  calDispType=Number  calEnum={'False', 'True'}  calGain=1.0  calOffset=0.0  calMax=inf  calMin=-inf  calFormat='-1'  calUnit=''  calHelp=''  calAccess=1  calFunction=[raptor_xcp_function(gcb) '|' raptor_get_param_eval(gcb, 'paramName') '_Override']
      settings: SourceProductName=Raptor
  raptor_override10 : Raptor_lib/Data Storage/raptor_override  paramName='Cal_A23_Duty'  nameSource=Parameter  measurement=None  calDispType=Number  calEnum={'False', 'True'}  calGain=1.0  calOffset=0.0  calMax=inf  calMin=-inf  calFormat='-1'  calUnit=''  calHelp=''  calAccess=1  calFunction=[raptor_xcp_function(gcb) '|' raptor_get_param_eval(gcb, 'paramName') '_Override']
      settings: SourceProductName=Raptor
  raptor_override11 : Raptor_lib/Data Storage/raptor_override  paramName='Cal_A93_Duty'  nameSource=Parameter  measurement=None  calDispType=Number  calEnum={'False', 'True'}  calGain=1.0  calOffset=0.0  calMax=inf  calMin=-inf  calFormat='-1'  calUnit=''  calHelp=''  calAccess=1  calFunction=[raptor_xcp_function(gcb) '|' raptor_get_param_eval(gcb, 'paramName') '_Override']
      settings: SourceProductName=Raptor
  raptor_override12 : Raptor_lib/Data Storage/raptor_override  paramName='Cal_K88_Duty'  nameSource=Parameter  measurement=None  calDispType=Number  calEnum={'False', 'True'}  calGain=1.0  calOffset=0.0  calMax=inf  calMin=-inf  calFormat='-1'  calUnit=''  calHelp=''  calAccess=1  calFunction=[raptor_xcp_function(gcb) '|' raptor_get_param_eval(gcb, 'paramName') '_Override']
      settings: SourceProductName=Raptor
  raptor_override3 : Raptor_lib/Data Storage/raptor_override  paramName='Cal_Water_Temp'  nameSource=Parameter  measurement=None  calDispType=Number  calEnum={'False', 'True'}  calGain=1.0  calOffset=0.0  calMax=inf  calMin=-inf  calFormat='-1'  calUnit=''  calHelp=''  calAccess=1  calFunction=[raptor_xcp_function(gcb) '|' raptor_get_param_eval(gcb, 'paramName') '_Override']
      settings: SourceProductName=Raptor
  raptor_override5 : Raptor_lib/Data Storage/raptor_override  paramName='Cal_Oil_Temp'  nameSource=Parameter  measurement=None  calDispType=Number  calEnum={'False', 'True'}  calGain=1.0  calOffset=0.0  calMax=inf  calMin=-inf  calFormat='-1'  calUnit=''  calHelp=''  calAccess=1  calFunction=[raptor_xcp_function(gcb) '|' raptor_get_param_eval(gcb, 'paramName') '_Override']
      settings: SourceProductName=Raptor
  raptor_override7 : Raptor_lib/Data Storage/raptor_override  paramName='Cal_OBU_Cooling_System_Output'  nameSource=Parameter  measurement=None  calDispType=Number  calEnum={'False', 'True'}  calGain=1.0  calOffset=0.0  calMax=inf  calMin=-inf  calFormat='-1'  calUnit=''  calHelp=''  calAccess=1  calFunction=[raptor_xcp_function(gcb) '|' raptor_get_param_eval(gcb, 'paramName') '_Override']
      settings: SourceProductName=Raptor
  raptor_table_1d5 : Raptor_lib/Table Lookup/raptor_table_1d  dataName='PW2PumpDuty'  initValue=|  dataType=double  storage=Calibration  initValueX=|  dataTypeXY=double  storageXY=Calibration  calVisible=on  showTable=on  calGain=1.0  calOffset=0.0  calMax=Inf  calMin=-Inf  calFormat='-1'  calUnit=''  calHelp=''  showBreakpoint=on  dataNameX=[]  calGainX=1.0  calOffsetX=0.0  calMaxX=Inf  calMinX=-Inf  calFormatX='-1'  calUnitX=''  calHelpX=''  calAccess=1  calFunction=raptor_xcp_function(gcb)  measureEnable=off  mName=[raptor_get_param_eval(gcb,'dataName'), '_Output']
      initValue=|
      | [10
      | 10
      | 20
      | 30
      | 40
      | 50
      | 60
      | 80
      | 100
      | 100
      | 100
      | ]
      initValueX=|
      | [0
      | 2.5
      | 5
      | 7.5
      | 10
      | 12.5
      | 15
      | 17.5
      | 20
      | 22.5
      | 25
      | ]
      settings: SourceProductName=Raptor
  raptor_table_1d7 : Raptor_lib/Table Lookup/raptor_table_1d  dataName='KY_Part_ADC2Degree'  initValue=|  dataType=double  storage=Calibration  initValueX=|  dataTypeXY=double  storageXY=Calibration  calVisible=on  showTable=on  calGain=1.0  calOffset=0.0  calMax=Inf  calMin=-Inf  calFormat='-1'  calUnit=''  calHelp=''  showBreakpoint=on  dataNameX=[]  calGainX=1.0  calOffsetX=0.0  calMaxX=Inf  calMinX=-Inf  calFormatX='-1'  calUnitX=''  calHelpX=''  calAccess=1  calFunction=raptor_xcp_function(gcb)  measureEnable=off  mName=[raptor_get_param_eval(gcb,'dataName'), '_Output']
      initValue=|
      | [0
      | 5
      | 10
      | 15
      | 20
      | 25
      | 30
      | 35
      | 40
      | 45
      | 50
      | 55
      | 60
      | 65
      | 70
      | 75
      | 80
      | 85
      | 90
      | 95
      | 100
      | 105
      | 110
      | 115
      | 120
      | 125
      | ]
      initValueX=|
      | [ 4.73 
      |  4.67 
      |  4.58 
      |  4.47 
      |  4.34 
      |  4.20 
      |  4.04 
      |  3.85 
      |  3.67 
      |  3.47 
      |  3.25 
      |  3.04 
      |  2.81 
      |  2.58 
      |  2.38 
      |  2.17 
      |  1.96 
      |  1.77 
      |  1.61 
      |  1.45 
      |  1.32 
      |  1.23 
      |  1.07 
      |  0.99 
      |  0.90 
      |  0.86 
      | ]
      settings: SourceProductName=Raptor
  wires:
  Demux2/2 -> raptor_override5/1, raptor_measurement2/1
  Demux2/1 -> raptor_override3/1, raptor_measurement3/1
  raptor_data_read7/1 -> Mux2/1
  Mux2/1 -> Gain4/1
  Gain4/1 -> Data Type Conversion2/1
  Data Type Conversion2/1 -> raptor_table_1d7/1
  raptor_table_1d7/1 -> Demux2/1
  raptor_data_read3/1 -> Mux2/2
  Relational Operator5/1 -> Delay2/1(Condition)
  raptor_adjustment8/1 -> Relational Operator5/2
  raptor_adjustment1/1 -> Relational Operator4/2
  raptor_adjustment13/1 -> Delay5/2(TimeCount)
  raptor_adjustment12/1 -> Delay2/2(TimeCount)
  raptor_override3/1 -> Relational Operator5/1, WC/1(WaterTemp), Relational Operator4/1
  Delay5/1(Output) -> Latch/1(Latch)
  Relational Operator4/1 -> Delay5/1(Condition)
  Delay2/1(Output) -> Latch/2(Reset)
  raptor_adjustment16/1 -> Relational Operator7/2
  Relational Operator6/1 -> Delay7/1(Condition)
  raptor_adjustment15/1 -> Relational Operator6/2
  raptor_adjustment14/1 -> Delay7/2(TimeCount)
  raptor_adjustment17/1 -> Delay6/2(TimeCount)
  raptor_override5/1 -> OC/1(WaterTemp), Relational Operator6/1, Relational Operator7/1
  Relational Operator7/1 -> Delay6/1(Condition)
  Delay7/1(Output) -> Latch1/1(Latch)
  Delay6/1(Output) -> Latch1/2(Reset)
  raptor_data_read2/1 -> Delay1/1(Condition), NOT/1
  Delay1/1(Output) -> Latch2/1(Latch)
  raptor_adjustment2/1 -> Delay1/2(TimeCount)
  raptor_adjustment3/1 -> Delay3/2(TimeCount)
  Delay3/1(Output) -> Latch2/2(Reset)
  NOT/1 -> Delay3/1(Condition)
  Latch2/1(Output) -> raptor_data_write2/1, raptor_data_write5/1
  Gain1/1 -> raptor_table_1d5/1
  raptor_table_1d5/1 -> OC/2(PW), WC/2(PW), AirC/2(PW)
  OC/1(Duty) -> raptor_override10/1
  raptor_override11/1 -> Mux1/1
  raptor_data_read5/1 -> Product5/1
  raptor_data_read10/1 -> Product5/2
  Product5/1 -> Gain1/1
  AirC/1(Duty) -> raptor_override12/1
  WC/1(Duty) -> raptor_override11/1
  raptor_data_read1/1 -> AirC/1(MaxTcell)
  raptor_data_read6/1 -> raptor_override1/1
  Constant/1 -> Subtract/1
  raptor_override10/1 -> Mux1/2
  Latch1/1(Output) -> Mux1/4
  Latch/1(Output) -> Mux1/3
  Data Type Conversion6/1 -> raptor_data_write8/1
  Data Type Conversion7/1 -> raptor_data_write9/1
  Mux1/1 -> Switch/1
  Switch/1 -> Demux1/1
  Demux1/1 -> Data Type Conversion7/1
  Demux1/3 -> Data Type Conversion/1
  Data Type Conversion/1 -> raptor_data_write1/1
  Demux1/4 -> Data Type Conversion5/1
  Data Type Conversion5/1 -> raptor_data_write6/1
  raptor_override1/1 -> Switch/2
  Demux1/2 -> Subtract1/2
  Subtract1/1 -> Data Type Conversion6/1
  Constant1/1 -> Subtract1/1
  raptor_override12/1 -> Switch1/1
  raptor_data_read8/1 -> raptor_override7/1
  raptor_override7/1 -> Switch1/2
  Switch1/1 -> Subtract/2
  Subtract/1 -> Data Type Conversion1/1
  Data Type Conversion1/1 -> raptor_data_write7/1

== system EPT/Foreground_TimeBase_5ms/System Initial ==
  Enable : EnablePort
  CAN_Setup_Related : Subsystem
  Constant : Constant  Value=0  OutDataTypeStr=boolean
  Constant2 : Constant  Value=5
  Data Type Conversion{1..2,4..5} (4 alike) : DataTypeConversion
  Delay : Delay  InitialCondition=0
  Delay1 : Subsystem
  Delay2 : Delay  InitialCondition=0
  Logical Operator : Logic  Inputs=3  AllPortsSameDT=off  OutDataTypeStr=boolean
  Mode_Related : Subsystem
  Motor_Related : Subsystem
  NOT : Logic  Operator=NOT  IconShape=distinctive  AllPortsSameDT=off  OutDataTypeStr=boolean
  PreCHG_Related : Subsystem
  Shutdown_Event_Related : Subsystem
  Shutdown_Event_Related1 : Subsystem
  Shutdown_Event_Related2 : Subsystem
  raptor_data_read : Raptor_lib/Data Storage/raptor_data_read  dataName='Flag_PowerOff_Finished'  dataShape=Scalar  idxSource=Input  idxRow=1  idxCol=1
      settings: SourceProductName=Raptor
  raptor_data_read1 : Raptor_lib/Data Storage/raptor_data_read  dataName='Fault_Reset_Trigger'  dataShape=Scalar  idxSource=Input  idxRow=1  idxCol=1
      settings: SourceProductName=Raptor
  raptor_data_write1 : Raptor_lib/Data Storage/raptor_data_write  dataName='LED_Status'  dataShape=Scalar  idxSource=Input Port  idxRow=1  idxCol=1
      settings: SourceProductName=Raptor
  raptor_data_write2 : Raptor_lib/Data Storage/raptor_data_write  dataName='Flag_SystemStart'  dataShape=Scalar  idxSource=Input Port  idxRow=1  idxCol=1
      settings: SourceProductName=Raptor
  raptor_data_write4 : Raptor_lib/Data Storage/raptor_data_write  dataName='A24_EOC_Enable'  dataShape=Scalar  idxSource=Input Port  idxRow=1  idxCol=1
      settings: SourceProductName=Raptor
  raptor_data_write5 : Raptor_lib/Data Storage/raptor_data_write  dataName='A10_CHG_Enable'  dataShape=Scalar  idxSource=Input Port  idxRow=1  idxCol=1
      settings: SourceProductName=Raptor
  wires:
  raptor_data_read/1 -> Logical Operator/2
  NOT/1 -> Logical Operator/1
  Logical Operator/1 -> Delay1/1(Condition)
  Delay/1 -> Delay2/1, Shutdown_Event_Related1/Trigger
  Delay1/1(Output) -> Delay/1, Shutdown_Event_Related/Trigger
  Delay2/1 -> Shutdown_Event_Related2/Trigger
  raptor_data_read1/1 -> Logical Operator/3
  Constant2/1 -> Delay1/2(TimeCount)
  Constant/1 -> Data Type Conversion4/1, PreCHG_Related/1(Init), CAN_Setup_Related/1(Init), NOT/1, Motor_Related/1(Init), Mode_Related/1(Init), Data Type Conversion2/1, Data Type Conversion1/1, Data Type Conversion5/1
  Data Type Conversion1/1 -> raptor_data_write1/1
  Data Type Conversion2/1 -> raptor_data_write2/1
  Data Type Conversion4/1 -> raptor_data_write4/1
  Data Type Conversion5/1 -> raptor_data_write5/1

== system EPT/Foreground_TimeBase_5ms/System Setup ==
  Enable : EnablePort
  "Dyno_Test " : Subsystem  Commented=on
  HV_Setup() : Subsystem
  Unit_Setup() : Subsystem

== system EPT/Foreground_TimeBase_5ms/SystemStart ==
  Trigger : TriggerPort  VariantControl=Variant  PortDimensions=1
  Constant : Constant  OutDataTypeStr=boolean
  raptor_data_def10 : Raptor_lib/Data Storage/raptor_data_def  dataName='Flag_SystemStart'  initValue=0  dataType=boolean  storage=Volatile (RAM)  calVisible=on  calType=Measurement  calDispType=Number  calEnum={'False', 'True'}  calGain=1.0  calOffset=0  calMin=-inf  calMax=inf  calFormat='-1'  calUnit=''  calHelp=''  calAccess=1  calFunction=raptor_xcp_function(gcb)  calDispHeaders=off  calColHeaders={'Col1' 'Col2' 'Col3'}  calRowHeaders={'Row1' 'Row2' 'Row3'}
      settings: SourceProductName=Raptor
  raptor_data_write1 : Raptor_lib/Data Storage/raptor_data_write  dataName='Flag_SystemStart'  dataShape=Scalar  idxSource=Input Port  idxRow=1  idxCol=1
      settings: SourceProductName=Raptor
  wires:
  Constant/1 -> raptor_data_write1/1

== system EPT/I//O/Application ==

== system EPT/I//O/Input ==
  ADC_ChargerPlugInterface : Subsystem
  "ADC_CoolingSystem " : Subsystem
  ADC_PlugOn : Subsystem
  ADC_Reserved : Subsystem
  ADC_TemperatureBatteryPack : Subsystem
  "Curtis_Reserved " : Subsystem
